simulink model "kalman"  (R2013b)
settings: Solver=ode3  StartTime=9  StopTime=57  FixedStep=0.1  RelTol=1e-3
settings Model: Creator=Franta  LastModifiedBy=Franta

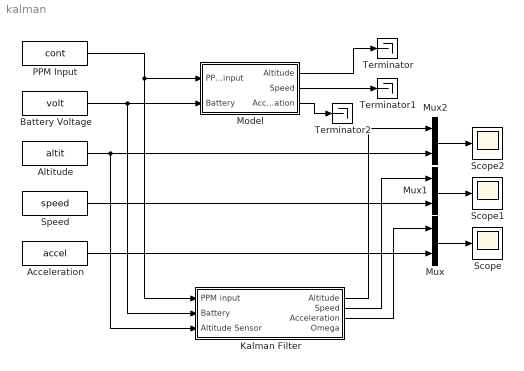
== system kalman ==
  Acceleration : FromWorkspace  VariableName=accel  SampleTime=0  OutputAfterFinalValue=Holding final value
  Altitude : FromWorkspace  VariableName=altit  SampleTime=0  OutputAfterFinalValue=Holding final value
  Battery Voltage : FromWorkspace  VariableName=volt  SampleTime=0  OutputAfterFinalValue=Holding final value
  Kalman Filter : Subsystem
  Model : Subsystem
  Mux : Mux  Inputs=2
  Mux1 : Mux  Inputs=2
  Mux2 : Mux  Inputs=2
  PPM Input : FromWorkspace  VariableName=cont  SampleTime=0  OutputAfterFinalValue=Holding final value
  Scope : Scope
      settings: YMin=0  YMax=47.5
  Scope1 : Scope
      settings: TimeRange=50
  Scope2 : Scope
      settings: SaveName=ScopeData2
  Speed : FromWorkspace  VariableName=speed  SampleTime=0  OutputAfterFinalValue=Holding final value
  Terminator : Terminator
  Terminator1 : Terminator
  Terminator2 : Terminator
  wires:
  Mux/1 -> Scope/1
  Mux1/1 -> Scope1/1
  Speed/1 -> Mux1/2
  Mux2/1 -> Scope2/1
  Acceleration/1 -> Mux/2
  PPM Input/1 -> Model/1(PPM input), Kalman Filter/1(PPM input)
  Battery Voltage/1 -> Kalman Filter/2(Battery), Model/2(Battery)
  Altitude/1 -> Kalman Filter/3(Altitude Sensor), Mux2/2
  Kalman Filter/1(Altitude) -> Mux2/1
  Kalman Filter/2(Speed) -> Mux1/1
  Kalman Filter/3(Acceleration) -> Mux/1
  Model/1(Altitude) -> Terminator/1
  Model/2(Speed) -> Terminator1/1
  Model/3(Acceleration) -> Terminator2/1

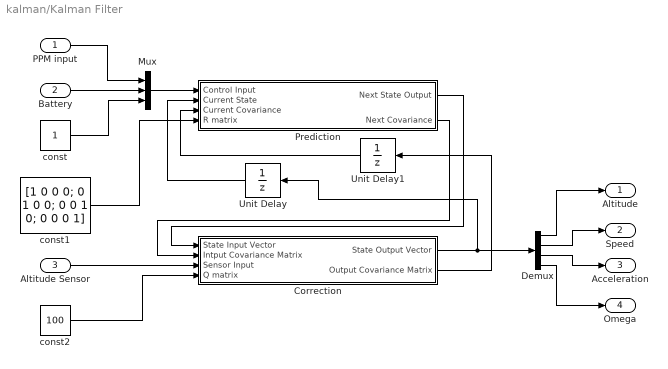
== system kalman/Kalman Filter ==
  PPM input : Inport
  Battery : Inport  Port=2
  Altitude Sensor : Inport  Port=3
  Correction : Subsystem
  Demux : Demux
  Mux : Mux  Inputs=3
  Prediction : Subsystem
  Unit Delay : UnitDelay  InitialCondition=[0 0 0 0]'  SampleTime=-1
  Unit Delay1 : UnitDelay  InitialCondition=[1 0 0 0; 0 1 0 0; 0 0 1 0; 0 0 0 1]  SampleTime=-1
  const : Constant
  const1 : Constant  Value=[1 0 0 0; 0 1 0 0; 0 0 1 0; 0 0 0 1]
  const2 : Constant  Value=100
  Altitude : Outport
  Speed : Outport  Port=2
  Acceleration : Outport  Port=3
  Omega : Outport  Port=4
  wires:
  Prediction/1(Next State Output) -> Correction/1(State Input Vector)
  Correction/1(State Output Vector) -> Demux/1, Unit Delay/1
  Correction/2(Output Covariance Matrix) -> Unit Delay1/1
  Mux/1 -> Prediction/1(Control Input)
  PPM input/1 -> Mux/1
  Battery/1 -> Mux/2
  const/1 -> Mux/3
  Altitude Sensor/1 -> Correction/3(Sensor Input)
  Demux/2 -> Speed/1
  Demux/3 -> Acceleration/1
  Demux/1 -> Altitude/1
  Demux/4 -> Omega/1
  Unit Delay/1 -> Prediction/2(Current State)
  Unit Delay1/1 -> Prediction/3(Current Covariance)
  Prediction/2(Next Covariance) -> Correction/2(Intput Covariance Matrix)
  const1/1 -> Prediction/4(R matrix)
  const2/1 -> Correction/4(Q matrix)

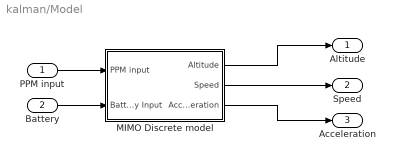
== system kalman/Model ==
  PPM input : Inport
  Battery : Inport  Port=2
  MIMO Discrete model : Subsystem
  Altitude : Outport
  Speed : Outport  Port=2
  Acceleration : Outport  Port=3
  wires:
  PPM input/1 -> MIMO Discrete model/1(PPM input)
  Battery/1 -> MIMO Discrete model/2(Battery Input)
  MIMO Discrete model/1(Altitude) -> Altitude/1
  MIMO Discrete model/2(Speed) -> Speed/1
  MIMO Discrete model/3(Acceleration) -> Acceleration/1

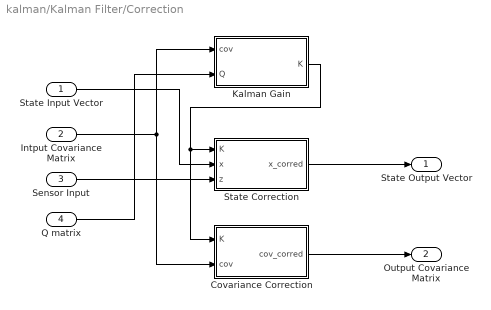
== system kalman/Kalman Filter/Correction ==
  State Input Vector : Inport
  Intput Covariance Matrix : Inport  Port=2
  Sensor Input : Inport  Port=3
  Q matrix : Inport  Port=4
  Covariance Correction : MATLAB Function  TreatAsAtomicUnit=on
  Kalman Gain : MATLAB Function  TreatAsAtomicUnit=on
  State Correction : MATLAB Function  TreatAsAtomicUnit=on
  State Output Vector : Outport
  Output Covariance Matrix : Outport  Port=2
  wires:
  Intput Covariance Matrix/1 -> Kalman Gain/1(cov), Covariance Correction/2(cov)
  Kalman Gain/1(K) -> Covariance Correction/1(K), State Correction/1(K)
  Sensor Input/1 -> State Correction/3(z)
  State Input Vector/1 -> State Correction/2(x)
  State Correction/1(x_corred) -> State Output Vector/1
  Covariance Correction/1(cov_corred) -> Output Covariance Matrix/1
  Q matrix/1 -> Kalman Gain/2(Q)

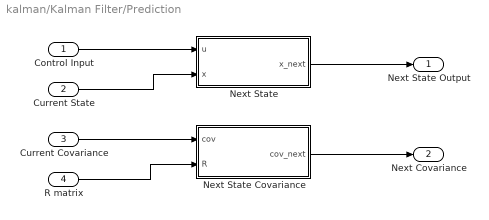
== system kalman/Kalman Filter/Prediction ==
  Control Input : Inport
  Current State : Inport  Port=2
  Current Covariance : Inport  Port=3
  R matrix : Inport  Port=4
  Next State : MATLAB Function  TreatAsAtomicUnit=on
  Next State Covariance : MATLAB Function  TreatAsAtomicUnit=on
  Next State Output : Outport
  Next Covariance : Outport  Port=2
  wires:
  Control Input/1 -> Next State/1(u)
  Current State/1 -> Next State/2(x)
  Current Covariance/1 -> Next State Covariance/1(cov)
  Next State/1(x_next) -> Next State Output/1
  Next State Covariance/1(cov_next) -> Next Covariance/1
  R matrix/1 -> Next State Covariance/2(R)

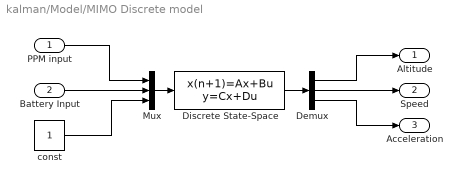
== system kalman/Model/MIMO Discrete model ==
  PPM input : Inport
  Battery Input : Inport  Port=2
  Demux : Demux  Outputs=3
  Discrete State-Space : DiscreteStateSpace  A=[1 0.1 0 0; 0 1 0.1 0; 0 0 0 1; 0 0 -0.6466 1.5736]  B=[0 0 0; 0 0 0; 0.002711 0.003372 -17.7363; 0.001897 0.08581 -13.3891]  C=[1 0 0 0; 0 1 0 0; 0 0 1 0]  D=[0 0 0; 0 0 0; 0 0 0]  SampleTime=0.1
  Mux : Mux  Inputs=3
  const : Constant
  Altitude : Outport
  Speed : Outport  Port=2
  Acceleration : Outport  Port=3
  wires:
  const/1 -> Mux/3
  Battery Input/1 -> Mux/2
  PPM input/1 -> Mux/1
  Discrete State-Space/1 -> Demux/1
  Demux/3 -> Acceleration/1
  Demux/2 -> Speed/1
  Demux/1 -> Altitude/1
  Mux/1 -> Discrete State-Space/1

== matlab function kalman/Kalman Filter/Prediction/Next State Covariance ==
  data: cov_next output; cov input; R input
function cov_next = nextstatecov(cov, R)
A = [1 0.1 0 0; 0 1 0.1 0; 0 0 0 1; 0 0 -0.6466 1.5736];

cov_next = (A*cov*A') + R;

== matlab function kalman/Kalman Filter/Prediction/Next State ==
  data: u input; x_next output; x input
function x_next = nextstate(u, x)
A = [1 0.1 0 0; 0 1 0.1 0; 0 0 0 1; 0 0 -0.6466 1.5736];
B = [0 0 0; 0 0 0; 0.002711 0.003372 -17.7363; 0.001897 0.08581 -13.3891];
x_next = A*x + B*u;

== matlab function kalman/Kalman Filter/Correction/Kalman Gain ==
  data: cov input; K output; Q input
function K = kalmangain(cov, Q)
P = [1 0 0 0];

K = (cov*P')/((P*cov*P') + Q);

== matlab function kalman/Kalman Filter/Correction/State Correction ==
  data: K input; x input; z input; x_corred output
function x_corred = stacorr(K, x, z)
P = [1 0 0 0];
x_corred = x + K*(z - P*x);

== matlab function kalman/Kalman Filter/Correction/Covariance Correction ==
  data: K input; cov input; cov_corred output
function cov_corred = covcorr(K, cov)
P = [1 0 0 0];
cov_corred = (diag([1 1 1 1]) - K*P)*cov;
